simulink model "continuous_triggered_subsystem"  (R2018a)
settings: Solver=VariableStepAuto  StartTime=0.0  StopTime=10.0  RelTol=1e-3
settings Model: Creator=BEAR  LastModifiedBy=BEAR

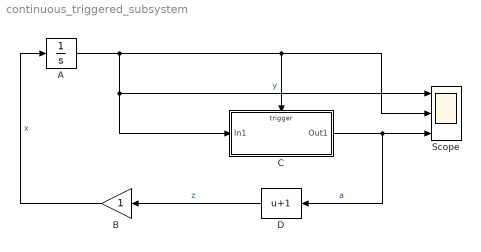
== system continuous_triggered_subsystem ==
  A : Integrator  InitialCondition=-1
  B : Gain  SampleTime=1
  C : Subsystem  TreatAsAtomicUnit=on
  D : Bias  Bias=1
  Scope : Scope  NumInputPorts=3
  wires:
  C/1(Out1) -> Scope/3, D/1  "a"
  A/1 -> Scope/2, C/Trigger, C/1(In1), Scope/1  "y"
  D/1 -> B/1  "z"
  B/1 -> A/1  "x"

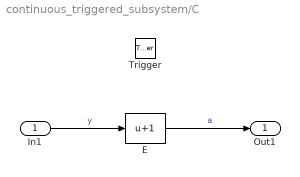
== system continuous_triggered_subsystem/C ==
  In1 : Inport
  Trigger : TriggerPort  VariantControl=Variant
  E : Bias  Bias=1
  Out1 : Outport
  wires:
  E/1 -> Out1/1  "a"
  In1/1 -> E/1  "y"
